simulink model "Controlador_Digital_Simulation_Espaco_de_Estados"  (R2017a)
settings: Solver=FixedStepAuto  StartTime=0.0  StopTime=0.2  FixedStep=1e-6  RelTol=1e-3
values from neighbouring files (symbols this model uses):
  A = [(-1/(C1*R6))                               1/(C1*R6)               0 ... (first row only)    [Controlador_Digital_Espaco_de_Estados.m]
  B = [    0 ... (first row only)    [Controlador_Digital_Espaco_de_Estados.m]
  C = [1, 0, 0]    [Controlador_Digital_Espaco_de_Estados.m]
  D = 0    [Controlador_Digital_Espaco_de_Estados.m]
  L = acker(A',C',Pl)'    [Controlador_Digital_Espaco_de_Estados.m]
  T = 2e-4    (= 0.0002)    [Controlador_Digital_Espaco_de_Estados.m]
undefined symbols (not defined in the file or in its folder): DiscIntNeverNeededParam, rank
libraries: fl_lib x20, nesl_utility x5, simulink x2
settings Model: Creator=Cleissom  LastModifiedBy=Cleissom

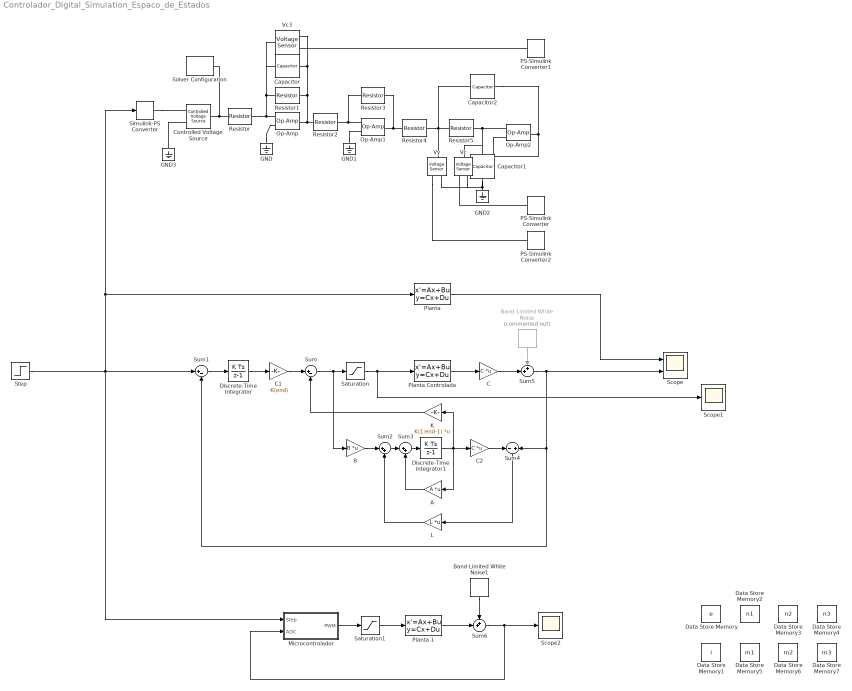
== system Controlador_Digital_Simulation_Espaco_de_Estados ==
  "A " : Gain  Gain=A  Multiplication=Matrix(K*u)
  B : Gain  Gain=B  Multiplication=Matrix(K*u)
  Band-Limited White Noise : simulink/Sources/Band-Limited White Noise  Commented=on  Cov=[0.00000003]  Ts=T  seed=[23341]
  Band-Limited White Noise1 : simulink/Sources/Band-Limited White Noise  Cov=[0.00000003]  Ts=T  seed=[23341]
  C : Gain  Gain=C  Multiplication=Matrix(K*u)
  C1 : Gain  Gain=-K(end)
  C2 : Gain  Gain=C  Multiplication=Matrix(K*u)
  Capacitor : fl_lib/Electrical/Electrical Elements/Capacitor  c=15 nF  r=1e-6 Ohm  g=0 1/Ohm  i_specify=off  i_priority=None  i=0 A  i_nominal_specify=off  i_nominal_unit=A  i_nominal_value=1  v_specify=off  v_priority=None  v=0 V  v_nominal_specify=off  v_nominal_unit=V  v_nominal_value=1  vc_specify=off  vc_priority=High  vc=0 V  vc_nominal_specify=off  vc_nominal_unit=V  vc_nominal_value=1
  Capacitor1 : fl_lib/Electrical/Electrical Elements/Capacitor  c=100 nF  r=1e-6 Ohm  g=0 1/Ohm  i_specify=off  i_priority=None  i=0 A  i_nominal_specify=off  i_nominal_unit=A  i_nominal_value=1  v_specify=off  v_priority=None  v=0 V  v_nominal_specify=off  v_nominal_unit=V  v_nominal_value=1  vc_specify=off  vc_priority=High  vc=0 V  vc_nominal_specify=off  vc_nominal_unit=V  vc_nominal_value=1
  Capacitor2 : fl_lib/Electrical/Electrical Elements/Capacitor  c=680 nF  r=1e-6 Ohm  g=0 1/Ohm  i_specify=off  i_priority=None  i=0 A  i_nominal_specify=off  i_nominal_unit=A  i_nominal_value=1  v_specify=off  v_priority=None  v=0 V  v_nominal_specify=off  v_nominal_unit=V  v_nominal_value=1  vc_specify=off  vc_priority=High  vc=0 V  vc_nominal_specify=off  vc_nominal_unit=V  vc_nominal_value=1
  Controlled Voltage Source : fl_lib/Electrical/Electrical Sources/Controlled Voltage Source
  Data Store Memory : DataStoreMemory  DataStoreName=e  ReadBeforeWriteMsg=warning  WriteAfterWriteMsg=warning  WriteAfterReadMsg=warning  ShowAdditionalParam=off  OutDataTypeStr=single
  Data Store Memory1 : DataStoreMemory  DataStoreName=i  ReadBeforeWriteMsg=warning  WriteAfterWriteMsg=warning  WriteAfterReadMsg=warning  ShowAdditionalParam=off  OutDataTypeStr=single
  Data Store Memory2 : DataStoreMemory  DataStoreName=n1  ReadBeforeWriteMsg=warning  WriteAfterWriteMsg=warning  WriteAfterReadMsg=warning  ShowAdditionalParam=off  OutDataTypeStr=single
  Data Store Memory3 : DataStoreMemory  DataStoreName=n2  ReadBeforeWriteMsg=warning  WriteAfterWriteMsg=warning  WriteAfterReadMsg=warning  ShowAdditionalParam=off  OutDataTypeStr=single
  Data Store Memory4 : DataStoreMemory  DataStoreName=n3  ReadBeforeWriteMsg=warning  WriteAfterWriteMsg=warning  WriteAfterReadMsg=warning  ShowAdditionalParam=off  OutDataTypeStr=single
  Data Store Memory5 : DataStoreMemory  DataStoreName=m1  ReadBeforeWriteMsg=warning  WriteAfterWriteMsg=warning  WriteAfterReadMsg=warning  ShowAdditionalParam=off  OutDataTypeStr=single
  Data Store Memory6 : DataStoreMemory  DataStoreName=m2  ReadBeforeWriteMsg=warning  WriteAfterWriteMsg=warning  WriteAfterReadMsg=warning  ShowAdditionalParam=off  OutDataTypeStr=single
  Data Store Memory7 : DataStoreMemory  DataStoreName=m3  ReadBeforeWriteMsg=warning  WriteAfterWriteMsg=warning  WriteAfterReadMsg=warning  ShowAdditionalParam=off  OutDataTypeStr=single
  Discrete-Time Integrator : DiscreteIntegrator  gainval=1  InitialConditionSetting=State (most efficient)  SampleTime=T  ICPrevOutput=DiscIntNeverNeededParam  ICPrevScaledInput=DiscIntNeverNeededParam
  Discrete-Time Integrator1 : DiscreteIntegrator  gainval=1  InitialConditionSetting=State (most efficient)  SampleTime=T  ICPrevOutput=DiscIntNeverNeededParam  ICPrevScaledInput=DiscIntNeverNeededParam
  GND{,1..3} (4 alike) : fl_lib/Electrical/Electrical Elements/Electrical Reference
  K : Gain  Gain=K(1:end-1)  Multiplication=Matrix(K*u)
  L : Gain  Gain=L  Multiplication=Matrix(K*u)
  Microcontrolador : MATLAB Function  TreatAsAtomicUnit=on  SystemSampleTime=T
  Op-Amp : fl_lib/Electrical/Electrical Elements/Op-Amp  outI_specify=off  outI_priority=None  outI=0 A  outI_nominal_specify=off  outI_nominal_unit=A  outI_nominal_value=1
  Op-Amp1 : fl_lib/Electrical/Electrical Elements/Op-Amp  outI_specify=off  outI_priority=None  outI=0 A  outI_nominal_specify=off  outI_nominal_unit=A  outI_nominal_value=1
  Op-Amp2 : fl_lib/Electrical/Electrical Elements/Op-Amp  outI_specify=off  outI_priority=None  outI=0 A  outI_nominal_specify=off  outI_nominal_unit=A  outI_nominal_value=1
  PS-Simulink Converter : nesl_utility/PS-Simulink Converter  PhysicalDomain=network_engine_domain  SubClassName=ps_output  LeftPortType=input  RightPortType=output  PseudoPeriodic=off  Frequencies=[]  Unit=1  AffineConversion=off
  PS-Simulink Converter1 : nesl_utility/PS-Simulink Converter  PhysicalDomain=network_engine_domain  SubClassName=ps_output  LeftPortType=input  RightPortType=output  PseudoPeriodic=off  Frequencies=[]  Unit=1  AffineConversion=off
  PS-Simulink Converter2 : nesl_utility/PS-Simulink Converter  PhysicalDomain=network_engine_domain  SubClassName=ps_output  LeftPortType=input  RightPortType=output  PseudoPeriodic=off  Frequencies=[]  Unit=1  AffineConversion=off
  "Planta " : StateSpace  A=A  B=B  C=C  D=D  X0=0
  Planta 1 : StateSpace  A=A  B=B  C=C  D=D  X0=0
  "Planta Controlada " : StateSpace  A=A  B=B  C=eye(rank(A))  D=zeros(rank(A),1);  X0=0
  Resistor{,1..3} (4 alike) : fl_lib/Electrical/Electrical Elements/Resistor  R=10 kOhm  i_specify=off  i_priority=None  i=0 A  i_nominal_specify=off  i_nominal_unit=A  i_nominal_value=1  v_specify=off  v_priority=None  v=0 V  v_nominal_specify=off  v_nominal_unit=V  v_nominal_value=1
  Resistor4 : fl_lib/Electrical/Electrical Elements/Resistor  R=68 kOhm  i_specify=off  i_priority=None  i=0 A  i_nominal_specify=off  i_nominal_unit=A  i_nominal_value=1  v_specify=off  v_priority=None  v=0 V  v_nominal_specify=off  v_nominal_unit=V  v_nominal_value=1
  Resistor5 : fl_lib/Electrical/Electrical Elements/Resistor  R=24 kOhm  i_specify=off  i_priority=None  i=0 A  i_nominal_specify=off  i_nominal_unit=A  i_nominal_value=1  v_specify=off  v_priority=None  v=0 V  v_nominal_specify=off  v_nominal_unit=V  v_nominal_value=1
  Saturation : Saturate  UpperLimit=3  LowerLimit=0
  Saturation1 : Saturate  UpperLimit=3  LowerLimit=0
  Scope : Scope  NumInputPorts=2
  Scope1 : Scope
  Scope2 : Scope
  Simulink-PS Converter : nesl_utility/Simulink-PS Converter  PhysicalDomain=network_engine_domain  SubClassName=ps_input  LeftPortType=input  RightPortType=output  PseudoPeriodic=off  Frequencies=[]  NoiseDistribution=none  NoiseParameters=[]  Unit=1  AffineConversion=off  FilteringAndDerivatives=provide  SimscapeFilterOrder=1  InputFilterTimeConstant=0.001  UdotUserProvided=0
  Solver Configuration : nesl_utility/Solver Configuration  PhysicalDomain=network_engine_domain  SubClassName=solver  LeftPortType=input  RightPortType=generic  Accelerate=off  Tones=[]  Harmonics=[]  SimulateNoise=off  Profile=off  UseLocalSampling=off  EnableSwitchedLinearOptims=on  FrequencyDomain=off  UseCCode=off  RelTol=0.001  AbsTol=1e-06  MinStep=1e-09  ToWorkspace=off  RevertToSquareIcSolve=off  NumHomotopyIterations=100  PhasorMode=off  PhasorModeNumHarmonics=1  OverrideAbsTol=off  DoDC=off  ResidualTolerance=1e-09  UseLocalSolver=off  LocalSolverChoice=NE_BACKWARD_EULER_ADVANCER  LocalSolverSampleTime=0.001  DoFixedCost=off  MaxNonlinIter=3  MaxModeIter=2  LinearAlgebra=Sparse  DelaysMemoryBudget=1024  AutomaticFiltering=on  FilteringTimeConstant=0.001
  Step : Step  Time=0  After=0.5  SampleTime=0
  Sum : Sum  Inputs=|+-
  Sum1 : Sum  Inputs=|+-
  Sum2 : Sum  Inputs=|++
  Sum3 : Sum  Inputs=|++
  Sum4 : Sum  Inputs=-|+
  Sum5 : Sum  Inputs=++|
  Sum6 : Sum  Inputs=++|
  Vc : fl_lib/Electrical/Electrical Sensors/Voltage Sensor
  Vc3 : fl_lib/Electrical/Electrical Sensors/Voltage Sensor
  Vy : fl_lib/Electrical/Electrical Sensors/Voltage Sensor
  wires:
  "Planta Controlada "/1 -> C/1
  Sum/1 -> B/1, Saturation/1
  Discrete-Time Integrator/1 -> C1/1
  C1/1 -> Sum/1
  Step/1 -> Microcontrolador/1(Step), Sum1/1, Simulink-PS Converter/1, "Planta "/1
  "A "/1 -> Sum3/2
  Sum4/1 -> L/1
  L/1 -> Sum2/2
  C2/1 -> Sum4/1
  Sum2/1 -> Sum3/1
  B/1 -> Sum2/1
  Discrete-Time Integrator1/1 -> "A "/1, K/1, C2/1
  K/1 -> Sum/2
  Sum1/1 -> Discrete-Time Integrator/1
  Sum3/1 -> Discrete-Time Integrator1/1
  Sum5/1 -> Sum4/2, Sum1/2, Scope/2
  C/1 -> Sum5/2
  Band-Limited White Noise/1 -> Sum5/1
  Saturation/1 -> Scope1/1, "Planta Controlada "/1
  "Planta "/1 -> Scope/1
  Microcontrolador/1(PWM) -> Saturation1/1
  Band-Limited White Noise1/1 -> Sum6/1
  Planta 1/1 -> Sum6/2
  Sum6/1 -> Microcontrolador/2(ADC), Scope2/1
  Saturation1/1 -> Planta 1/1
  connections:
  Resistor1/LConn1 -- Vc3/LConn1 -- Capacitor/LConn1 -- Resistor/RConn1 -- Op-Amp/LConn2
  Capacitor/RConn1 -- Resistor1/RConn1 -- Resistor2/LConn1 -- Op-Amp/RConn1 -- Vc3/RConn2
  Resistor2/RConn1 -- Resistor3/LConn1 -- Op-Amp1/LConn2
  GND/LConn1 -- Op-Amp/LConn1
  Resistor3/RConn1 -- Resistor4/LConn1 -- Op-Amp1/RConn1
  Op-Amp1/LConn1 -- GND1/LConn1
  Resistor4/RConn1 -- Capacitor2/LConn1 -- Resistor5/LConn1 -- Vy/LConn1
  Resistor5/RConn1 -- Vc/LConn1 -- Capacitor1/LConn1 -- Op-Amp2/LConn1
  Op-Amp2/RConn1 -- Capacitor2/RConn1 -- Op-Amp2/LConn2
  GND2/LConn1 -- Vc/RConn2 -- Vy/RConn2 -- Capacitor1/RConn1
  Simulink-PS Converter/RConn1 -- Controlled Voltage Source/RConn1
  Controlled Voltage Source/LConn1 -- Solver Configuration/RConn1 -- Resistor/LConn1
  GND3/LConn1 -- Controlled Voltage Source/RConn2
  PS-Simulink Converter/LConn1 -- Vc/RConn1
  PS-Simulink Converter1/LConn1 -- Vc3/RConn1
  Vy/RConn1 -- PS-Simulink Converter2/LConn1

== matlab function Controlador_Digital_Simulation_Espaco_de_Estados/Microcontrolador ==
  data: Step input; ADC input; PWM output; e data_store_memory; i data_store_memory; n2 data_store_memory; n1 data_store_memory; n3 data_store_memory; m1 data_store_memory; m2 data_store_memory; m3 data_store_memory
function PWM = fcn(Step, ADC)


A           = single([-416.67, 416.67, 0; -355.39, 333.77, 21.626; 0, 0, -6666.7]);
B3          = single(6666.7);

K           = single([-0.99525, 2.106, -0.86308, 106.05]);

L           = single([13165, 1.1583e+05, -2.5599]);

Ts          = single(0.0002);

%%

global i
global e
global n1
global n2
global n3
global m1
global m2
global m3

%%

rawValue = single((4095*ADC)/3.3);  % Converte valor de tensão para variável

c = single((4499*rawValue)/4095);   % Converte para o domínio de Pulso

setValue = single((4499*Step)/3.3);

enew = setValue - c;
inew = (Ts*e + i);

n1new = (Ts*m1 + n1);
n2new = (Ts*m2 + n2);
n3new = (Ts*m3 + n3);

k = (K(1)*n1new + K(2)*n2new + K(3)*n3new);
x = (inew*K(4) - k);

PWM = double((3.3*x)/4499); % Converte do domínio do Pulso para Tensão

m1 = single((c-n1new)*L(1) + (n1new*A(1,1)) + (n2new*A(1,2)) + (n3new*A(1,3)));
m2 = single((c-n1new)*L(2) + (n1new*A(2,1)) + (n2new*A(2,2)) + (n3new*A(2,3)));
m3 = single((c-n1new)*L(3) + (n1new*A(3,1)) + (n2new*A(3,2)) + (n3new*A(3,3)) + x*B3);

e = enew;
i = inew;
n1 = n1new;
n2 = n2new;
n3 = n3new;

test = double([enew]);
